simulink model "full_sys1"  (R2022a)
settings: Solver=FixedStepAuto  StartTime=0.0  StopTime=10.0  RelTol=1e-3  EnableMultiTasking=on
libraries: mbedblockslib x25, simulink x6, hdlsllib x6
(part 2 of 2)

== system full_sys1/Subsystem/System Update and Heirarchy/Alarm Prioritize ==
  note: Create final ALARM message
  note: What if BOTH ? - consecutive
  note: Single byte Alert:
      | UPPER 4-bits:
      | 0x10 - Power
      | 0x20 - Alarm
      | 0x30 - Pressure
      | 0x40 - Flow...
      |
      | LOWER 4-bits:
      | over/under/bat_%/time_out
  note: Remove this whole block and forward Alarm Codes directly
  note: Alarm Alerts:
      | 0x21 - No Alarm
      | 0x22 - Over_Time
  note: PSU Alerts:
      | 0x11 - Normal (AC)
      | 0x12 - Battery 75%
      | 0x13 - Battery 50%
      | 0x14 - Battery 25%
  P_Alrm : Inport
  A_Alrm : Inport  Port=2
  Alarm Alert : Subsystem  TreatAsAtomicUnit=on
  Data Type Conversion : DataTypeConversion  OutDataTypeStr=double  SaturateOnIntegerOverflow=off  RndMeth=Floor
  Display : Display
  Display1 : Display
  Display2 : Display
  If : If  NumInputs=2  IfExpression=(u1 > 17)  ElseIfExpressions=(u2 > 33)
  Merge : Merge  Inputs=3
  No_Alarm1 : Subsystem  TreatAsAtomicUnit=on
  Power Alert : Subsystem  TreatAsAtomicUnit=on
  ALRM_Out : Outport
  wires:
  P_Alrm/1 -> Data Type Conversion/1, Display/1, If/1
  A_Alrm/1 -> Display1/1, If/2
  If/1 -> Power Alert/Action
  Merge/1 -> Display2/1, ALRM_Out/1
  Power Alert/1(Out1) -> Merge/1
  Alarm Alert/1(Out1) -> Merge/2
  No_Alarm1/1(Out1) -> Merge/3
  Data Type Conversion/1 -> Power Alert/1(P_Alrm)
  If/2 -> Alarm Alert/Action
  If/3 -> No_Alarm1/Action

== system full_sys1/Subsystem/System Update and Heirarchy/Array Index Get ==
  note: Get byte[0]
  note: Extract Specific Byte from HMI_Input Array
  note: Get byte[1]
  Usr_In : Inport
  Constant1 : Constant
  Constant2 : Constant  Value=0
  Display1 : Display
  Display12 : Display
  Display4 : Display
  Index Vector : MultiPortSwitch  DataPortOrder=Zero-based contiguous  Inputs=1  zeroidx=on  SaturateOnIntegerOverflow=off  InputSameDT=off
  Index Vector1 : MultiPortSwitch  DataPortOrder=Zero-based contiguous  Inputs=1  zeroidx=on  SaturateOnIntegerOverflow=off  InputSameDT=off
  HMI_Cmd1 : Outport
  New_Val1 : Outport  Port=2
  wires:
  Index Vector/1 -> HMI_Cmd1/1, Display4/1
  Constant2/1 -> Index Vector/1
  Usr_In/1 -> Display12/1, Index Vector1/2, Index Vector/2
  Constant1/1 -> Index Vector1/1
  Index Vector1/1 -> New_Val1/1, Display1/1

== system full_sys1/Subsystem/System Update and Heirarchy/Power_CMD ==
  note: REMOVED PSU CHECK (ALARM & HMI WILL CHECK)
  note: PASS PSU CODE DIRECTLY
  note: 0x14 = 20dec
  note: (PSU)
      | Read Sub-System Status Commands
      | Normal operation = No 2nd byte
      | Event trigger (2) = DC voltage forwarded
  note: Get Lower 4 bits
  note: Battery Status:
      | 0x10 - AC
      | 0x11 - 75%
      | 0x12 - 50%
      | 0x13 - 25%
  note: PSU Alerts:
      | 0x11 - Normal (AC)
      | 0x12 - Battery 75%
      | 0x13 - Battery 50%
      | 0x14 - Battery 25%
  note: Error Code (99)
  P_Cmd : Inport
  AC POWER : Subsystem  Commented=on  TreatAsAtomicUnit=on
  Bitwise Operator1 : simulink/Logic and Bit Operations/Bitwise Operator  Commented=on  logicop=AND  UseBitMask=on  BitMask=bin2dec('00001111')  BitMaskRealWorld=Stored Integer
  Constant : Constant  Commented=on  Value=0x13
  Constant2 : Constant  Commented=on  Value=0x14  SampleTime=-1
  Constant3 : Constant  Commented=on  Value=0x63  SampleTime=-1
  DC POWER : Subsystem  Commented=on  TreatAsAtomicUnit=on
  Display1 : Display  Commented=on
      settings: Format=hex (Stored Integer)
  ERROR MSG1 : Subsystem  Commented=on  TreatAsAtomicUnit=on
  Merge1 : Merge  Commented=on  Inputs=4
  Power_Other : Subsystem  Commented=on  TreatAsAtomicUnit=on
  Switch Case1 : SwitchCase  Commented=on  CaseConditions={0x01, 0x02, 0x03}
  P_Alrm : Outport
  wires:
  Switch Case1/4 -> ERROR MSG1/Action
  Constant2/1 -> Power_Other/1(In1)
  Switch Case1/1 -> AC POWER/Action
  Switch Case1/3 -> Power_Other/Action
  Bitwise Operator1/1 -> Switch Case1/1
  Switch Case1/2 -> DC POWER/Action
  Constant3/1 -> ERROR MSG1/1(In1)
  Power_Other/1(Out1) -> Merge1/3
  ERROR MSG1/1(Out1) -> Merge1/4
  AC POWER/1(Out1) -> Merge1/1
  DC POWER/1(DC_out) -> Merge1/2
  P_Cmd/1 -> P_Alrm/1
  Constant/1 -> DC POWER/1(DC_in), Bitwise Operator1/1
  Merge1/1 -> Display1/1

== system full_sys1/Subsystem/System Update and Heirarchy/Update Internal Variables ==
  note: 'GoTo' Output variables
      | (motor control etc.)
  note: Update the system variable with User_Input
      | Save new value to correct
      | Array element for system update
  note: Variables:
      | [0] - CPAP
      | [1] - EPAP
      | [2] - IPAP
      | [3] - FiO2
      | [4] - APNEA
  note: Array Element
  note: Value to be stored
  note: Should be from updated HMI
      | Input Value Array[0-4] .
      | Single value at the moment.
  note: 'GoTo' Motor Controller Block
  HMI_Cmd1 : Inport
  New_Val1 : Inport  Port=2
  Display : Display
  Display1 : Display
  Display2 : Display
  HMI_CMD1 : Subsystem
  Subsystem : Subsystem
  tag scope: sys_var=global
  wires:
  HMI_CMD1/1(Element1) -> Display/1, Subsystem/1(Element1)
  HMI_Cmd1/1 -> HMI_CMD1/1(H_Cmd)
  New_Val1/1 -> [sys_var], Subsystem/2(Value1), Display1/1
  Subsystem/1(Var_Arr) -> Display2/1

== system full_sys1/Subsystem/Sensor_Monitor/Flow1_Monitor/Hi_Alert1 ==
  note: If within normal pressure range,
      | forward that value to HMI for display
  note: Above FlowRate threshold = 0x42
  note: 0x42 = 66 dec
  note: Above Flow Rate (1) Threshold
  Action Port : ActionPort  ActionPortLabel=elseif((u1 >= 80))
  Alert1 : Constant  Value=66
  Out1 : Outport
  wires:
  Alert1/1 -> Out1/1

== system full_sys1/Subsystem/Sensor_Monitor/Flow1_Monitor/Lo_Alert1 ==
  note: Below Flow Rate (1) Threshold
  note: Below FlowRate Threshold = 0x43
  note: 0x43 = 67 dec
  Action Port : ActionPort  ActionPortLabel=if((u1 <= 10))
  Alert1 : Constant  Value=67
  Out1 : Outport
  wires:
  Alert1/1 -> Out1/1

== system full_sys1/Subsystem/Sensor_Monitor/Flow1_Monitor/No_Alert1 ==
  note: No Alert (normal range) = 0x01
  note: 0x41 = 65 dec
  note: Within Flow Rate (1) Threshold
  Action Port : ActionPort  ActionPortLabel=else
  Alert1 : Constant  Value=65
  no_v : Outport
  wires:
  Alert1/1 -> no_v/1

== system full_sys1/Subsystem/Sensor_Monitor/Flow2_Monitor/Hi_Alert2 ==
  note: If within normal pressure range,
      | forward that value to HMI for display
  note: Above FlowRate threshold = 0x42
  note: 0x62 = 98 dec
  note: Below Flow Rate (2) Threshold
  Action Port : ActionPort  ActionPortLabel=elseif((u1 >= 80))
  Alert1 : Constant  Value=98
  Out1 : Outport
  wires:
  Alert1/1 -> Out1/1

== system full_sys1/Subsystem/Sensor_Monitor/Flow2_Monitor/Lo_Alert2 ==
  note: Below Flow Rate (2) Threshold
  note: Below FlowRate Threshold = 0x43
  note: 0x63 = 99 dec
  Action Port : ActionPort  ActionPortLabel=if((u1 <= 10))
  Alert1 : Constant  Value=99
  Out1 : Outport
  wires:
  Alert1/1 -> Out1/1

== system full_sys1/Subsystem/Sensor_Monitor/Flow2_Monitor/No_Alert2 ==
  note: No Alert (normal range) = 0x01
  note: 0x61 = 97 dec
  note: Within Flow Rate (2) Threshold
  Action Port : ActionPort  ActionPortLabel=else
  Alert1 : Constant  Value=97
  no_v : Outport
  wires:
  Alert1/1 -> no_v/1

== system full_sys1/Subsystem/Sensor_Monitor/Pressure1_Monitor/Hi_Alert1 ==
  note: Above Pressure threshold
  note: 0x32 = 50 dec
  note: Above Pressure Threshold = 0x32
  Action Port : ActionPort  ActionPortLabel=elseif((u1 >= 20))
  Alert1 : Constant  Value=50
  Out1 : Outport
  wires:
  Alert1/1 -> Out1/1

== system full_sys1/Subsystem/Sensor_Monitor/Pressure1_Monitor/Lo_Alert1 ==
  note: 0x33 = 51 dec
  note: Below Pressure Threshold = 0x33
  Action Port : ActionPort  ActionPortLabel=if((u1 <= 5))
  Alert1 : Constant  Value=51
  Out1 : Outport
  wires:
  Alert1/1 -> Out1/1

== system full_sys1/Subsystem/Sensor_Monitor/Pressure1_Monitor/No_Alert1 ==
  note: No Trigger - Within Range
  note: No Alert (normal range)
  note: If within normal pressure range,
      | forward that value to HMI for display
  note: 0x31 - 49 dec
  Action Port : ActionPort  ActionPortLabel=else
  Alert1 : Constant  Value=49
  no_v : Outport
  wires:
  Alert1/1 -> no_v/1

== system full_sys1/Subsystem/Sensor_Monitor/Pressure2_Monitor/Hi_Alert1 ==
  note: Above Pressure threshold
  note: 0x52 = 82 dec
  note: Above Pressure (2) Threshold = 0x52
  Action Port : ActionPort  ActionPortLabel=elseif((u1 >= 20))
  Alert1 : Constant  Value=82
  Out1 : Outport
  wires:
  Alert1/1 -> Out1/1

== system full_sys1/Subsystem/Sensor_Monitor/Pressure2_Monitor/Lo_Alert1 ==
  note: 0x53 = 83 dec
  note: Below Pressure (2) Threshold = 0x53
  Action Port : ActionPort  ActionPortLabel=if((u1 <= 5))
  Alert1 : Constant  Value=83
  Out1 : Outport
  wires:
  Alert1/1 -> Out1/1

== system full_sys1/Subsystem/Sensor_Monitor/Pressure2_Monitor/No_Alert1 ==
  note: No Trigger - Within Range
  note: No Alert (normal range)
  note: If within normal pressure range,
      | forward that value to HMI for display
  note: 0x31 - 49 dec
  Action Port : ActionPort  ActionPortLabel=else
  Alert1 : Constant  Value=49
  no_v : Outport
  wires:
  Alert1/1 -> no_v/1

== system full_sys1/Subsystem/Sensor_Monitor/Subsystem/FiO2_Alert ==
  note: Pressure Alert
  FiO2_Alrm : Inport
  Action Port : ActionPort  ActionPortLabel=elseif( (u5 >= 114))
  Out1 : Outport
  wires:
  FiO2_Alrm/1 -> Out1/1

== system full_sys1/Subsystem/Sensor_Monitor/Subsystem/Flow_Alert1 ==
  note: Either Pressure OR Power Alert!
  F1_Alrm : Inport
  Action Port : ActionPort  ActionPortLabel=elseif((u2 >= 66))
  Out1 : Outport
  wires:
  F1_Alrm/1 -> Out1/1

== system full_sys1/Subsystem/Sensor_Monitor/Subsystem/Flow_Alert2 ==
  note: Pressure Alert
  F2_Alrm : Inport
  Action Port : ActionPort  ActionPortLabel=elseif( (u4 >= 98))
  Out1 : Outport
  wires:
  F2_Alrm/1 -> Out1/1

== system full_sys1/Subsystem/Sensor_Monitor/Subsystem/No_Alert ==
  note: 0X01 = NO ALERTS
  note: Normal Opertaion (No Alerts)
  Action Port : ActionPort  ActionPortLabel=else
  Constant : Constant  Value=33
  Out1 : Outport
  wires:
  Constant/1 -> Out1/1

== system full_sys1/Subsystem/Sensor_Monitor/Subsystem/Press_Alert1 ==
  note: Pressure Alert
  P1_Alrm : Inport
  Action Port : ActionPort  ActionPortLabel=if((u1 >= 50))
  Out1 : Outport
  wires:
  P1_Alrm/1 -> Out1/1

== system full_sys1/Subsystem/Sensor_Monitor/Subsystem/Press_Alert2 ==
  note: Pressure (2) High or Low
  P2_Alrm : Inport
  Action Port : ActionPort  ActionPortLabel=elseif( (u3 >= 82))
  Out1 : Outport
  wires:
  P2_Alrm/1 -> Out1/1

== system full_sys1/Subsystem/Sub-Systems Read/REMOVE/Signal Increment ==
  note: If 2nd byte received?
      | Then clear counter?
  HMI_Msg : Inport
  Data Store Memory : DataStoreMemory  DataStoreName=Cnt1  WriteAfterWriteMsg=warning  InitialValue=-1  ShowAdditionalParam=off
  Data Store Read : DataStoreRead  DataStoreName=Cnt1  IndexOptions=Index vector (dialog)  Indices=1  OutputSizes=1
  Data Store Write : DataStoreWrite  DataStoreName=Cnt1  IndexOptions=Index vector (dialog)  Indices=1  OutputSizes=1
  Display : Display
  If : If  IfExpression=(u1 > 1)
  Merge : Merge
  Normal : Subsystem  TreatAsAtomicUnit=on
  if_counter : Subsystem  TreatAsAtomicUnit=on
  H_Byt : Outport
  wires:
  If/1 -> if_counter/Action
  Normal/1(no_v) -> Merge/2
  if_counter/1(Out1) -> Merge/1
  If/2 -> Normal/Action
  Data Store Read/1 -> if_counter/1(cnt)
  HMI_Msg/1 -> If/1
  Merge/1 -> Display/1, Data Store Write/1, H_Byt/1

== system full_sys1/Subsystem/Sub-Systems Read/REMOVE/Subsystem ==
  note: Update single element of input array
  Value1 : Inport
  Element1 : Inport  Port=2
  Assignment : Assignment  IndexMode=Zero-based  DiagnosticForDimensions=Warning  IndexOptions=Index vector (port)  Indices=0  OutputSizes=1
  Constant3 : Constant  Value=[0, 0]
  Data Type Conversion1 : DataTypeConversion  OutDataTypeStr=uint8  SaturateOnIntegerOverflow=off  RndMeth=Floor
  H_Cmd : Outport
  wires:
  Value1/1 -> Assignment/2
  Assignment/1 -> H_Cmd/1
  Data Type Conversion1/1 -> Assignment/1
  Constant3/1 -> Data Type Conversion1/1
  Element1/1 -> Assignment/3

== system full_sys1/Subsystem/Sub-Systems Write/Combine All/Hi_Alert1 ==
  note: Sensor Alerts Take Lowest Priority
  AlmSNS : Inport
  Action Port : ActionPort  ActionPortLabel=elseif((u2 >= 20))
  Out1 : Outport
  wires:
  AlmSNS/1 -> Out1/1

== system full_sys1/Subsystem/Sub-Systems Write/Combine All/Hi_Alert2 ==
  note: 0x21 = 33 dec
  note: If No Alert
  Action Port : ActionPort  ActionPortLabel=else
  No Alert1 : Constant  Value=33
  Out1 : Outport
  wires:
  No Alert1/1 -> Out1/1

== system full_sys1/Subsystem/Sub-Systems Write/Combine All/Lo_Alert1 ==
  note: Sub-System Alert Take Highest Priority
  AlmSBS : Inport
  Action Port : ActionPort  ActionPortLabel=if((u1 > 33))
  Out1 : Outport
  wires:
  AlmSBS/1 -> Out1/1

== system full_sys1/Subsystem/Sub-Systems Write/Combine All/Subsystem3 ==
  note: Need Global Array??
  note: Update single element of input array
  Index1 : Inport
  Sense1 : Inport  Port=2
  Array : Inport  Port=3
  Assignment : Assignment  IndexMode=Zero-based  DiagnosticForDimensions=Warning  IndexOptions=Index vector (port)  Indices=0  OutputSizes=1
  Flow2 : Outport
  wires:
  Index1/1 -> Assignment/3
  Sense1/1 -> Assignment/2
  Assignment/1 -> Flow2/1
  Array/1 -> Assignment/1

== system full_sys1/Subsystem/System Update and Heirarchy/Alarm Prioritize/Alarm Alert ==
  note: 0x22 = 34 dec
  note: ALARM OVER 2 MINUTES
  Action Port : ActionPort  ActionPortLabel=elseif((u2 > 33))
  Constant : Constant  Value=34
  Out1 : Outport
  wires:
  Constant/1 -> Out1/1

== system full_sys1/Subsystem/System Update and Heirarchy/Alarm Prioritize/No_Alarm1 ==
  note: Normal Opertaion (No Alerts)
  Action Port : ActionPort  ActionPortLabel=else
  Constant : Constant  Value=33
  Out1 : Outport
  wires:
  Constant/1 -> Out1/1

== system full_sys1/Subsystem/System Update and Heirarchy/Alarm Prioritize/Power Alert ==
  note: Battery Alert & Capacity in same byte
  note: PSU Power Alert + Battery %
  P_Alrm : Inport
  Action Port : ActionPort  ActionPortLabel=if((u1 > 17))
  Out1 : Outport
  wires:
  P_Alrm/1 -> Out1/1

== system full_sys1/Subsystem/System Update and Heirarchy/Power_CMD/AC POWER ==
  Action Port : ActionPort
  Constant : Constant  Value=0x10
  Out1 : Outport
  wires:
  Constant/1 -> Out1/1

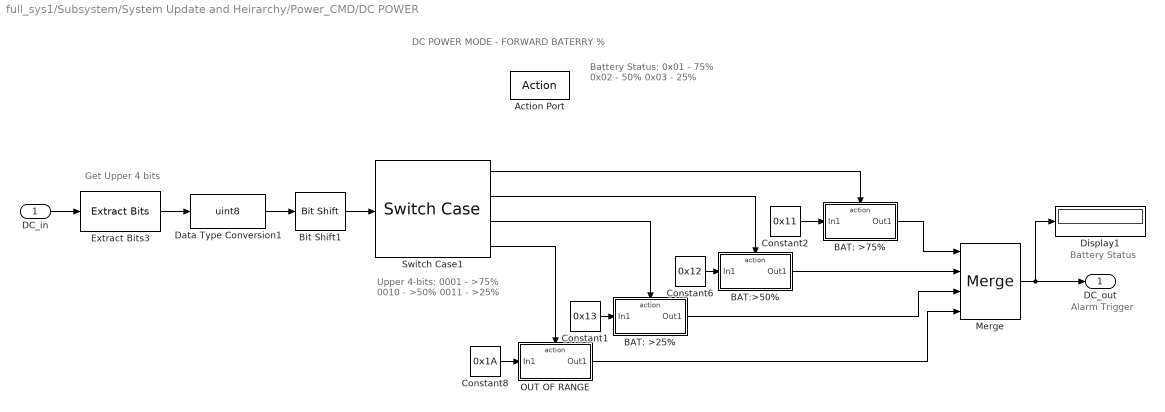
== system full_sys1/Subsystem/System Update and Heirarchy/Power_CMD/DC POWER ==
  note: Battery Status
  note: Upper 4-bits:
      | 0001 - >75%
      | 0010 - >50%
      | 0011 - >25%
  note: DC POWER MODE - FORWARD BATERRY %
  note: Get Upper 4 bits
  note: Alarm Trigger
  note: Battery Status:
      | 0x01 - 75%
      | 0x02 - 50%
      | 0x03 - 25%
  DC_in : Inport
  Action Port : ActionPort
  BAT: >25% : Subsystem  TreatAsAtomicUnit=on
  BAT: >75% : Subsystem  TreatAsAtomicUnit=on
  BAT:>50% : Subsystem  TreatAsAtomicUnit=on
  Bit Shift1 : hdlsllib/Logic and Bit Operations/Bit Shift  mode=Shift Right Logical  N=4
  Constant1 : Constant  Value=0x13  SampleTime=-1
  Constant2 : Constant  Value=0x11  SampleTime=-1
  Constant6 : Constant  Value=0x12  SampleTime=-1
  Constant8 : Constant  Value=0x1A  SampleTime=-1
  Data Type Conversion1 : DataTypeConversion  OutDataTypeStr=uint8  SaturateOnIntegerOverflow=off  RndMeth=Floor
  Display1 : Display
      settings: Format=hex (Stored Integer)
  Extract Bits3 : simulink/Logic and Bit Operations/Extract Bits  bitsToExtract=Upper half  numBits=8  bitIdxRange=[0 7]  outScalingMode=Preserve fixed-point scaling
  Merge : Merge  Inputs=4
  OUT OF RANGE : Subsystem  TreatAsAtomicUnit=on
  Switch Case1 : SwitchCase  CaseConditions={0x01, 0x02, 0x03}
  DC_out : Outport
  wires:
  Switch Case1/3 -> BAT: >25%/Action
  Merge/1 -> DC_out/1, Display1/1
  Constant8/1 -> OUT OF RANGE/1(In1)
  OUT OF RANGE/1(Out1) -> Merge/4
  BAT: >75%/1(Out1) -> Merge/1
  Extract Bits3/1 -> Data Type Conversion1/1
  Switch Case1/2 -> BAT:>50%/Action
  Bit Shift1/1 -> Switch Case1/1
  BAT:>50%/1(Out1) -> Merge/2
  Constant6/1 -> BAT:>50%/1(In1)
  Data Type Conversion1/1 -> Bit Shift1/1
  BAT: >25%/1(Out1) -> Merge/3
  Switch Case1/4 -> OUT OF RANGE/Action
  Switch Case1/1 -> BAT: >75%/Action
  Constant2/1 -> BAT: >75%/1(In1)
  Constant1/1 -> BAT: >25%/1(In1)
  DC_in/1 -> Extract Bits3/1

== system full_sys1/Subsystem/System Update and Heirarchy/Power_CMD/ERROR MSG1 ==
  In1 : Inport
  Action Port : ActionPort
  Out1 : Outport
  wires:
  In1/1 -> Out1/1

== system full_sys1/Subsystem/System Update and Heirarchy/Power_CMD/Power_Other ==
  note: Do what with each
      | Triggerd bit?
  In1 : Inport
  Action Port : ActionPort
  Out1 : Outport
  wires:
  In1/1 -> Out1/1

== system full_sys1/Subsystem/System Update and Heirarchy/Update Internal Variables/HMI_CMD1 ==
  note: 51=H33
  note: was arr[5]
  note: Create 2 more cases:
      | Case[3] update system array
      | Case[5] updates ALARM
      | Case[9] updates MODE
  note: (HMI)
      | Read Sub-System Status Commands
  note: Get Lower 4 bits
  note: MSG (lower):
      | 0x01 - Normal Op
      | 0x03 - User Input
      | 0x05 - Alarm Silence
      | 0x09 - Mode
  H_Cmd : Inport
  Bitwise Operator : simulink/Logic and Bit Operations/Bitwise Operator  logicop=AND  UseBitMask=on  BitMask=bin2dec('00001111')  BitMaskRealWorld=Stored Integer
  Constant5 : Constant  Value=0
  Display : Display
  Display1 : Display
  ERROR MSG : Subsystem  TreatAsAtomicUnit=on
  EVENT TRGR : Subsystem  TreatAsAtomicUnit=on
  Merge2 : Merge  Inputs=3
  NO USER_IN : Subsystem  TreatAsAtomicUnit=on
  Switch Case : SwitchCase  CaseConditions={0x01, [0x03, 0x05, 0x09]}
  Element1 : Outport
  wires:
  ERROR MSG/1(Out1) -> Merge2/3
  Constant5/1 -> ERROR MSG/1(In1)
  Bitwise Operator/1 -> Switch Case/1, Display1/1
  Switch Case/2 -> EVENT TRGR/Action
  NO USER_IN/1(Out1) -> Merge2/1
  Switch Case/1 -> NO USER_IN/Action
  Switch Case/3 -> ERROR MSG/Action
  EVENT TRGR/1(Arr1) -> Merge2/2
  Merge2/1 -> Element1/1
  H_Cmd/1 -> EVENT TRGR/1(H_Cmd), Bitwise Operator/1, Display/1

== system full_sys1/Subsystem/System Update and Heirarchy/Update Internal Variables/Subsystem ==
  note: System Array
      | 5 Value to track
  note: Update specific single element of input array
  note: Global Array to update internal (local) system variables
      | Use 'GoTo' & 'From' to pass newly updated variable to Output Block
  Element1 : Inport
  Value1 : Inport  Port=2
  Assignment : Assignment  IndexMode=Zero-based  DiagnosticForDimensions=Warning  IndexOptions=Index vector (port)  Indices=0  OutputSizes=1
  Constant3 : Constant  Value=[0, 0, 0, 0, 0]
  Data Type Conversion1 : DataTypeConversion  OutDataTypeStr=uint8  SaturateOnIntegerOverflow=off  RndMeth=Floor
  Var_Arr : Outport
  wires:
  Value1/1 -> Assignment/2
  Assignment/1 -> Var_Arr/1
  Data Type Conversion1/1 -> Assignment/1
  Constant3/1 -> Data Type Conversion1/1
  Element1/1 -> Assignment/3

== system full_sys1/Subsystem/Sub-Systems Read/REMOVE/Signal Increment/Normal ==
  note: Normal HMI - Clear Counter
  Action Port : ActionPort
  Constant : Constant  Value=0
  no_v : Outport
  wires:
  Constant/1 -> no_v/1

== system full_sys1/Subsystem/Sub-Systems Read/REMOVE/Signal Increment/if_counter ==
  note: was if(u1>2)
  note: Byte Counter Handler
  note: Increment Counter
  note: If (counter >2) {Clear}
  cnt : Inport
  Action Port : ActionPort
  Add : Sum
  Constant : Constant
  If : If  IfExpression=u1 >= 2
  Merge : Merge
  clear_cnt : Subsystem  TreatAsAtomicUnit=on
  count : Subsystem  TreatAsAtomicUnit=on
  Out1 : Outport
  wires:
  cnt/1 -> Add/1
  Constant/1 -> Add/2
  If/1 -> clear_cnt/Action
  clear_cnt/1(Out1) -> Merge/1
  count/1(no_v) -> Merge/2
  If/2 -> count/Action
  Add/1 -> count/1(cnt), If/1
  Merge/1 -> Out1/1

== system full_sys1/Subsystem/System Update and Heirarchy/Power_CMD/DC POWER/BAT: >25% ==
  In1 : Inport
  Action Port : ActionPort
  Out1 : Outport
  wires:
  In1/1 -> Out1/1

== system full_sys1/Subsystem/System Update and Heirarchy/Power_CMD/DC POWER/BAT: >75% ==
  In1 : Inport
  Action Port : ActionPort
  Out1 : Outport
  wires:
  In1/1 -> Out1/1

== system full_sys1/Subsystem/System Update and Heirarchy/Power_CMD/DC POWER/BAT:>50% ==
  In1 : Inport
  Action Port : ActionPort
  Out1 : Outport
  wires:
  In1/1 -> Out1/1

== system full_sys1/Subsystem/System Update and Heirarchy/Power_CMD/DC POWER/OUT OF RANGE ==
  In1 : Inport
  Action Port : ActionPort
  Out1 : Outport
  wires:
  In1/1 -> Out1/1

== system full_sys1/Subsystem/System Update and Heirarchy/Update Internal Variables/HMI_CMD1/ERROR MSG ==
  In1 : Inport
  Action Port : ActionPort  ActionPortLabel=default:
  Out1 : Outport
  wires:
  In1/1 -> Out1/1

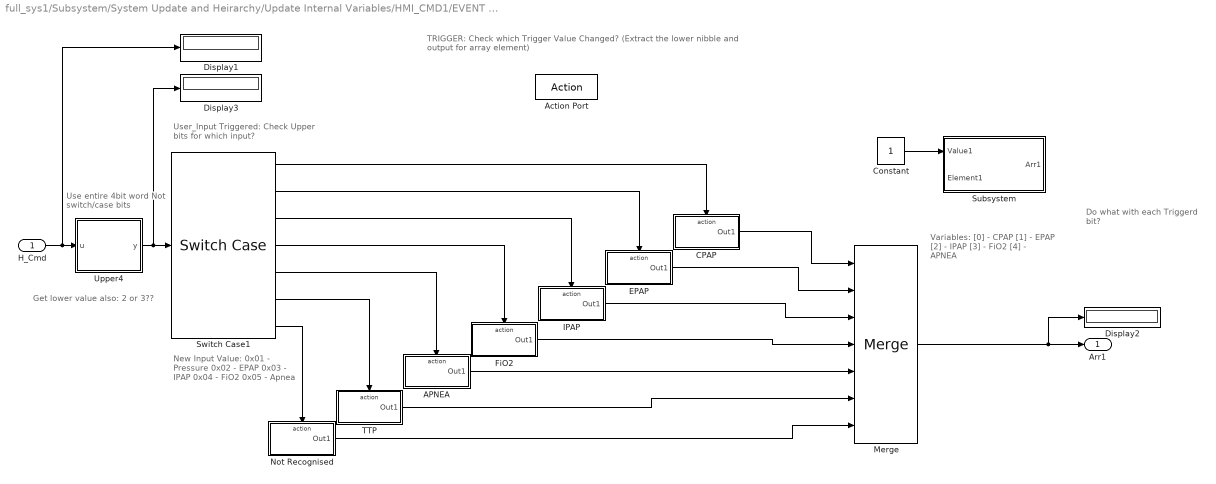
== system full_sys1/Subsystem/System Update and Heirarchy/Update Internal Variables/HMI_CMD1/EVENT TRGR ==
  note: TRIGGER: Check which Trigger Value Changed?
      | (Extract the lower nibble and output for array element)
  note: User_Input Triggered:
      | Check Upper bits for which input?
  note: Use entire 4bit word
      | Not switch/case bits
  note: Do what with each
      | Triggerd bit?
  note: New Input Value:
      | 0x01 - Pressure
      | 0x02 - EPAP
      | 0x03 - IPAP
      | 0x04 - FiO2
      | 0x05 - Apnea
  note: Get lower value also: 2 or 3??
  note: Variables:
      | [0] - CPAP
      | [1] - EPAP
      | [2] - IPAP
      | [3] - FiO2
      | [4] - APNEA
  H_Cmd : Inport
  Action Port : ActionPort  ActionPortLabel=case [ 3 5 9 ]:
  APNEA : Subsystem  TreatAsAtomicUnit=on
  CPAP : Subsystem  TreatAsAtomicUnit=on
  Constant : Constant
  Display1 : Display
  Display2 : Display
  Display3 : Display
  EPAP : Subsystem  TreatAsAtomicUnit=on
  FiO2 : Subsystem  TreatAsAtomicUnit=on
  IPAP : Subsystem  TreatAsAtomicUnit=on
  Merge : Merge  Inputs=7
  Not Recognised : Subsystem  TreatAsAtomicUnit=on
  Subsystem : Subsystem
  Switch Case1 : SwitchCase  CaseConditions={0x00, 0x01, 0x02, 0x03, 0x04, 0x05}
  TTP : Subsystem  TreatAsAtomicUnit=on
  Upper4 : Subsystem
  Arr1 : Outport
  wires:
  Switch Case1/2 -> EPAP/Action
  Switch Case1/1 -> CPAP/Action
  Switch Case1/7 -> Not Recognised/Action
  CPAP/1(Out1) -> Merge/1
  EPAP/1(Out1) -> Merge/2
  Not Recognised/1(Out1) -> Merge/7
  Switch Case1/3 -> IPAP/Action
  Switch Case1/4 -> FiO2/Action
  IPAP/1(Out1) -> Merge/3
  FiO2/1(Out1) -> Merge/4
  H_Cmd/1 -> Display1/1, Upper4/1(u)
  Upper4/1(y) -> Display3/1, Switch Case1/1
  Constant/1 -> Subsystem/1(Value1)
  Switch Case1/5 -> APNEA/Action
  Switch Case1/6 -> TTP/Action
  Merge/1 -> Display2/1, Arr1/1
  APNEA/1(Out1) -> Merge/5
  TTP/1(Out1) -> Merge/6

== system full_sys1/Subsystem/System Update and Heirarchy/Update Internal Variables/HMI_CMD1/NO USER_IN ==
  note: No User_Input from HMI - Do nothing
      | Continue Normal Operation
  note: was arr[5]
  Action Port : ActionPort  ActionPortLabel=case [ 1 ]:
  Constant5 : Constant  Value=0
  Out1 : Outport
  wires:
  Constant5/1 -> Out1/1

== system full_sys1/Subsystem/Sub-Systems Read/REMOVE/Signal Increment/if_counter/clear_cnt ==
  note: Clear Counter
  Action Port : ActionPort
  Constant : Constant  Value=-1
  Out1 : Outport
  wires:
  Constant/1 -> Out1/1

== system full_sys1/Subsystem/Sub-Systems Read/REMOVE/Signal Increment/if_counter/count ==
  note: Continue Counter
  cnt : Inport
  Action Port : ActionPort
  no_v : Outport
  wires:
  cnt/1 -> no_v/1

== system full_sys1/Subsystem/System Update and Heirarchy/Update Internal Variables/HMI_CMD1/EVENT TRGR/APNEA ==
  note: APNEA
  Action Port : ActionPort  ActionPortLabel=case [ 4 ]:
  Constant : Constant  Value=4
  Out1 : Outport
  wires:
  Constant/1 -> Out1/1

== system full_sys1/Subsystem/System Update and Heirarchy/Update Internal Variables/HMI_CMD1/EVENT TRGR/CPAP ==
  Action Port : ActionPort  ActionPortLabel=case [ 0 ]:
  Constant : Constant  Value=0
  Out1 : Outport
  wires:
  Constant/1 -> Out1/1

== system full_sys1/Subsystem/System Update and Heirarchy/Update Internal Variables/HMI_CMD1/EVENT TRGR/EPAP ==
  note: EPAP
  Action Port : ActionPort  ActionPortLabel=case [ 1 ]:
  Constant : Constant
  Out1 : Outport
  wires:
  Constant/1 -> Out1/1

== system full_sys1/Subsystem/System Update and Heirarchy/Update Internal Variables/HMI_CMD1/EVENT TRGR/FiO2 ==
  note: FiO2
  Action Port : ActionPort  ActionPortLabel=case [ 3 ]:
  Constant : Constant  Value=3
  Out1 : Outport
  wires:
  Constant/1 -> Out1/1

== system full_sys1/Subsystem/System Update and Heirarchy/Update Internal Variables/HMI_CMD1/EVENT TRGR/IPAP ==
  note: IPAP
  Action Port : ActionPort  ActionPortLabel=case [ 2 ]:
  Constant : Constant  Value=2
  Out1 : Outport
  wires:
  Constant/1 -> Out1/1

== system full_sys1/Subsystem/System Update and Heirarchy/Update Internal Variables/HMI_CMD1/EVENT TRGR/Not Recognised ==
  note: Must be within array element range [0-3]
  Action Port : ActionPort  ActionPortLabel=default:
  Constant : Constant  Value=0
  Out1 : Outport
  wires:
  Constant/1 -> Out1/1

== system full_sys1/Subsystem/System Update and Heirarchy/Update Internal Variables/HMI_CMD1/EVENT TRGR/Subsystem ==
  note: Update single element of input array
  Value1 : Inport
  Element1 : Inport  Port=2
  Assignment : Assignment  IndexMode=Zero-based  DiagnosticForDimensions=Warning  IndexOptions=Index vector (port)  Indices=0  OutputSizes=1
  Constant5 : Constant  Value=[0,0,0,0]
  Arr1 : Outport
  wires:
  Constant5/1 -> Assignment/1
  Value1/1 -> Assignment/2
  Element1/1 -> Assignment/3
  Assignment/1 -> Arr1/1

== system full_sys1/Subsystem/System Update and Heirarchy/Update Internal Variables/HMI_CMD1/EVENT TRGR/TTP ==
  note: Time To Peak
  Action Port : ActionPort  ActionPortLabel=case [ 5 ]:
  Constant : Constant  Value=5
  Out1 : Outport
  wires:
  Constant/1 -> Out1/1

== system full_sys1/Subsystem/System Update and Heirarchy/Update Internal Variables/HMI_CMD1/EVENT TRGR/Upper4 ==
  note: Get Upper 4 bits
  u : Inport
  Bit Shift1 : hdlsllib/Logic and Bit Operations/Bit Shift  mode=Shift Right Logical  N=4
  Data Type Conversion1 : DataTypeConversion  OutDataTypeStr=uint8  SaturateOnIntegerOverflow=off  RndMeth=Floor
  Extract Bits3 : simulink/Logic and Bit Operations/Extract Bits  bitsToExtract=Upper half  numBits=8  bitIdxRange=[0 7]  outScalingMode=Preserve fixed-point scaling
  y : Outport
  wires:
  Data Type Conversion1/1 -> Bit Shift1/1
  Bit Shift1/1 -> y/1
  Extract Bits3/1 -> Data Type Conversion1/1
  u/1 -> Extract Bits3/1

== stateflow chart full_sys1/Subsystem/Proportional (mass) Flow Control/Chart ==
  note: Same value follower code as Motor Controller
      | Except keep within 20% - 100% Oxygen (FiO2)?
  state Parent1
    state Master1
      entry:
      LED = 1; % visual
      Digital = 1; %activate
      exit:
    state Master2
      entry:
      data = 0x55; % 30%
      exit:
    state Master3
      entry:
      LED = 0; % visual
      exit:
    (default) -> Master1
    Master1 -> Master2 : after(2,sec)
    Master2 -> Master3 : after(2,sec)
  state Parent2
    state Master4
      entry:
      LED = 1; % visual
      Digital = 1; %activate
      exit:
    state Master5
      entry:
      data = 0xB2; % 70%
      exit:
    state Master6
      entry:
      LED = 0; % visual
      exit:
    (default) -> Master4
    Master4 -> Master5 : after(2,sec)
    Master5 -> Master6 : after(2,sec)
  note: Keep range of [30% - 70%]
  note: 0xC0 = 3/4 Vout
      | 0xB2 = 70% Vout
      | 0x80 = 1/2 Vout
      | 0x55 = 30% Vout
      | 0x40 = 1/4 Vout
  (default) -> Parent1
  Parent1 -> Parent2 : after(6,sec)
  Parent2 -> Parent1 : after(6,sec)
  data: data output; LED output; Digital output; input input

== stateflow chart full_sys1/Subsystem/Motor Controller/Chart ==
  state MOTOR
    note: Unused for now...
    note: Adjust according to User Value?
    state SHUTDOWN % Blower Off
      state Stop_1 % I2C to Anal.
        entry:
        speed = 0x00; % slowest?
        %LED = 1;
        exit:
      state Stop_2 % Motor Brake
        entry:
        mtr_brk = 0; % Enable
        %LED = 0; % debug
        exit:
      state Stop_3 % Motor Disable
        entry:
        mtr_dis = 0; % Disable
        %LED = 1; % debug
        exit:
      state Stop_4 % Main Power
        entry:
        mtr_pwr = 0; % OFF
        % LED = 0; % debug
        exit:
      (default) -> Stop_1 % I2C to Anal.
      Stop_1 % I2C to Anal. -> Stop_2 % Motor Brake : after(2,sec)
      Stop_2 % Motor Brake -> Stop_3 % Motor Disable : after(2,sec)
      Stop_3 % Motor Disable -> Stop_4 % Main Power : after(2,sec)
    state STARTUP % Blower Start
      state Start_1 % Main Power
        entry:
        mtr_pwr = 1; % ON
        %LED = 1; % debug
        exit:
      state Start_2 % Motor Brake
        entry:
        mtr_brk = 1; % Disable
        mtr_dis = 1; % Enabled
        %LED = 0; % debug
        exit:
      (default) -> Start_1 % Main Power
      Start_1 % Main Power -> Start_2 % Motor Brake : after(1,sec)
    state PID % Adjust 10 time per sec?
      note: User Range:
          | max = 20
          | min = 4
      state PID_1
        entry: temp = 10;
        % Start in the middle
        speed = temp;
        exit:
      note: Speed Values:
          | 0xA0 = 3/4 Vout
          | 0x80 = 1/2 Vout
          | 0x40 = 1/4 Vout
      note: Pressure Range:
          | max = +61mBar
          | 0 = 1mBar
          | min = -61mBar
      state PID_2
        entry:
        % slow value follwer
        speed = temp;
        exit:
      state Decrement1
        entry:
        if(speed > 10)
        temp = speed - 5;
        end
        exit:
      state Increment
        entry:
        if(speed < 250)
        temp = speed + 5;
        end
        exit:
      (default) -> PID_1
      PID_1 -> PID_2 : after(100,msec)
      Decrement1 -> PID_2 : after(50,msec)
      Increment -> PID_2 : after(50,msec)
      PID_2 -> (junction 67)
      (junction 67) -> (junction 69)
      (junction 69) -> Increment [order 1] : [pressure < user_in]
      (junction 69) -> Decrement1 [order 2] : [pressure > user_in]
    note: 1. Power - On
        | 2. Brake - Off
        | 3. Disable - Off
        | 4. Voltage Output
    note: BRAKE PIN:
        | Enabled = <0.8V or Gnd
        | Deactivated = >2.4V or Not wired
    note: DISABLE PIN:
        | Disable = <0.8V or Gnd
        | Enable = >2.4V or Not wired
    note: "speed" must increase/decrease until "pressure" = "user_in"
    note: Compensate for negative pressures (-61 -> 0)
    note: NOTE:
        | * Large step sizes - Shift values faster
        | * Small step sizes - Closer to required value
    (default) -> STARTUP % Blower Start
    STARTUP % Blower Start -> PID % Adjust 10 time per sec? : after(2,sec)
    PID % Adjust 10 time per sec? -> SHUTDOWN % Blower Off : after(120, sec)
  (default) -> MOTOR
  data: speed output; mtr_brk output; mtr_pwr output; mtr_dis output; pressure input; user_in input; power input; temp local uint8

== stateflow chart full_sys1/Subsystem/Pressure_Sensor_1/Testing/Chart1 ==
  state entry_
    if(hmi < 62)
    display = hmi;
    else % Positive-Negative
    display = hmi - 255;
    end
  (default) -> entry_
  data: hmi input; display output

== stateflow chart full_sys1/Subsystem/Proportional (mass) Flow Control/Chart1 ==
  state MOTOR
    note: Adjust according to User Value?
    note: Unused for now...
    state STARTUP % Flow_Ctrl Start
      state Start_1 % Main Power
        entry:
        mtr_pwr = 1; % ON
        %LED = 1; % debug
        exit:
      state Start_2 % Motor Brake
        entry:
        mtr_brk = 1; % Disable
        %LED = 0; % debug
        exit:
      (default) -> Start_1 % Main Power
      Start_1 % Main Power -> Start_2 % Motor Brake : after(1,sec)
    state PID % Adjust 10 time per sec?
      note: User Range:
          | max = 20
          | min = 4
      state PID_1
        entry: temp = 10;
        % Start in the middle
        speed = temp;
        exit:
      note: Speed Values:
          | 0xA0 = 3/4 Vout
          | 0x80 = 1/2 Vout
          | 0x40 = 1/4 Vout
      note: Pressure Range:
          | max = +61mBar
          | 0 = 1mBar
          | min = -61mBar
      state PID_2
        entry:
        % slow value follwer
        speed = temp;
        exit:
      state Decrement1
        entry: LED = 0;
        if(speed > 10)
        temp = speed - 5;
        end
        exit:
      state Increment
        entry: LED = 1;
        if(speed < 250)
        temp = speed + 5;
        end
        exit:
      (default) -> PID_1
      PID_1 -> PID_2 : after(100,msec)
      Decrement1 -> PID_2 : after(50,msec)
      Increment -> PID_2 : after(50,msec)
      PID_2 -> (junction 67)
      (junction 67) -> (junction 69)
      (junction 69) -> Increment [order 1] : [pressure < user_in]
      (junction 69) -> Decrement1 [order 2] : [pressure > user_in]
    state SHUTDOWN % Blower Off
      state Stop_1 % I2C to Anal.
        entry:
        speed = 0x00; % slowest?
        LED = 1;
        exit:
      state Stop_2 % Motor Brake
        entry:
        mtr_brk = 0; % Enable
        LED = 0; % debug
        exit:
      state Stop_3 % Motor Disable
        entry:
        mtr_dis = 0; % Disable
        LED = 1; % debug
        exit:
      state Stop_4 % Main Power
        entry:
        mtr_pwr = 0; % OFF
        LED = 0; % debug
        exit:
      (default) -> Stop_1 % I2C to Anal.
      Stop_1 % I2C to Anal. -> Stop_2 % Motor Brake : after(2,sec)
      Stop_2 % Motor Brake -> Stop_3 % Motor Disable : after(2,sec)
      Stop_3 % Motor Disable -> Stop_4 % Main Power : after(2,sec)
    note: 1. Power - On
        | 2. Brake - Off
        | 3. Disable - Off
        | 4. Voltage Output
    note: BRAKE PIN:
        | Enabled = <0.8V or Gnd
        | Deactivated = >2.4V or Not wired
    note: DISABLE PIN:
        | Disable = <0.8V or Gnd
        | Enable = >2.4V or Not wired
    note: "speed" must increase/decrease until "pressure" = "user_in"
    note: Compensate for negative pressures (-61 -> 0)
    note: NOTE:
        | * Large step sizes - Shift values faster
        | * Small step sizes - Closer to required value
    (default) -> (junction 47)
    (junction 47) -> (junction 48) [order 2]
    (junction 47) -> STARTUP % Flow_Ctrl Start [order 1] : [power == 1]
    (junction 48) -> SHUTDOWN % Blower Off
    STARTUP % Flow_Ctrl Start -> PID % Adjust 10 time per sec? : after(2,sec)
  (default) -> MOTOR
  data: speed output; LED output; mtr_brk output; mtr_pwr output; mtr_dis output; pressure input; user_in input; power input; temp local uint8

== stateflow chart full_sys1/Subsystem/Motor Controller/LED ==
  note: TEST:
      | Routine Checks
  state Run % Parent
    state Check % Check Sub-Systems
      entry:
      LED = 0; % LED Off
      exit:
    state LED % Child
      entry: % none
      LED = 1; % LED On
      exit: % none
    (default) -> LED % Child
    LED % Child -> Check % Check Sub-Systems : after(2,sec)
    Check % Check Sub-Systems -> LED % Child : after(2,sec)
  note: Check Input
      | Power present?
  (default) -> Run % Parent
  data: LED output

== stateflow chart full_sys1/Subsystem/Pressure_Sensor_1/Testing/Chart ==
  state Pos_Neg
    entry:
    if(sensor >= 0)
    trans = sensor;
    %elseif(sensor == -0)
    %   trans = 1;
    else % negative to Positive
    trans = 255 + sensor;
    end
  (default) -> Pos_Neg
  data: sensor input; trans output
